simulink model "sampleModel1826"  (R2023a)
settings: Solver=VariableStepAuto  StartTime=0.0  StopTime=10.0  RelTol=1e-3
libraries: hdlsllib x4
settings Model: Creator=user1  LastModifiedBy=user1

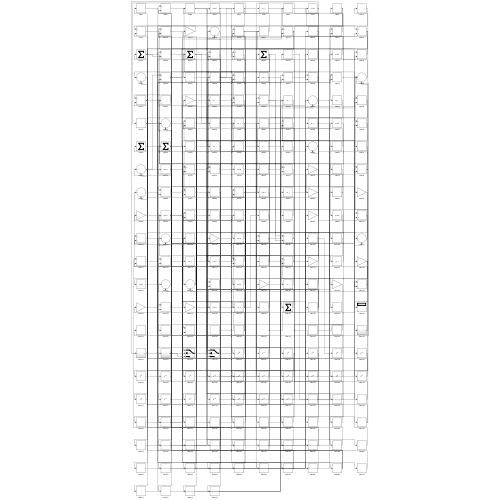
[thumbnail: Simulink's stored preview of the top-level diagram]
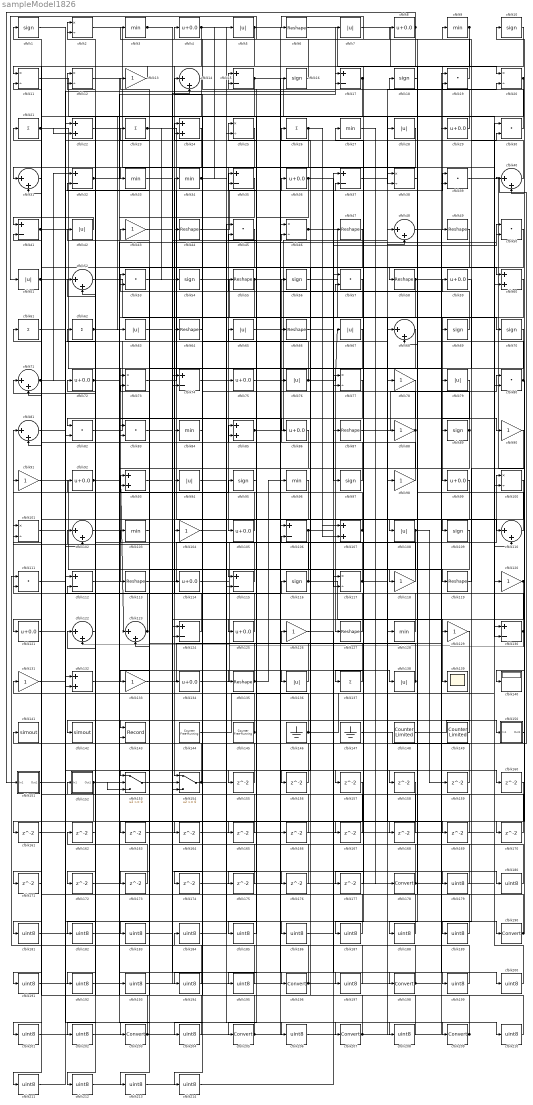
== system sampleModel1826 ==
  cfblk{1,10,16,18,54,56,69..70,89,95,97,109,116} (13 alike) : Signum
  cfblk{2,11..12,20,25,38,46,73,77,100..101,117} (12 alike) : Product  Inputs=*/  RndMeth=Zero  SaturateOnIntegerOverflow=on
  cfblk{14,31,40,48,52,68,71,81,102,110,122..123} (12 alike) : Sum  Inputs=|++
  cfblk{3,9,27,33..34,84,96,103,128} (9 alike) : MinMax
  cfblk{13,43,78,88,90..91,98,104,118,120,126,129,131,133} (14 alike) : Gain
  cfblk{4,8,29,36,59,72,75,86,92,99,105,114,121,125,134} (15 alike) : Bias  Bias=0.0  SaturateOnIntegerOverflow=off
  cfblk{15,17,32,35,37,41,74,106,112,115,124,130} (12 alike) : Sum  Inputs=+-
  cfblk{22,24,60,85,93,107,132} (7 alike) : Sum
  cfblk{5,7,28,42,51,63,65,67,76,79,94,108,136,138} (14 alike) : Abs  SaturateOnIntegerOverflow=off
  cfblk{19,30,39,45,50,53,57,80,82..83,111} (11 alike) : DotProduct  OutDataTypeStr=Inherit: Inherit via internal rule
  cfblk{6,44,47,49,55,58,64,66,87,113,119,127,135} (13 alike) : Reshape
  cfblk{21,23,26,61..62,137} (6 alike) : Sum  Inputs=+
  cfblk139 : Scope
  cfblk140 : Display
  cfblk141 : ToWorkspace  VariableName=simout  SaveFormat=Timeseries  SampleTime=-1
  cfblk142 : ToWorkspace  VariableName=simout  SaveFormat=Timeseries  SampleTime=-1
  cfblk143 : Record  FileSettingsInternal="{\"entries\":[{\"content\":{\"excelSettings\":{\"content\":{},\"type\":\"Streamout.ExcelSettings\"}},\"type\":\"Streamout.FileSettingStorage\",\"uuid\":\"\"}],\"packageUris\":[\"http:\\/\\/schema.mathworks.com\\/mf0\\/streamout_blocks\\/R2020a\"],\"version\":\"1.0\"}"  Layout=[1 1]  SignalsInternal="{\"entries\":[{\"content\":{\"signals\":[{\"content\":{\"blockPath\":[],\"dimensions\":[1],\"domain\":\"\",\"lineColor\":\"#a2142f\",\"plots\":[1],\"port\":1,\"signalID\":4356,\"signalName\":\"XY Graph:1\"},\"type\":\"RecordBlkView.Signal\",\"uuid\":\"\"},{\"content\":{\"blockPath\":[],\"dimensions\":[1],\"domain\":\"\",\"lineColor\":\"#139fff\",\"plots\":[1],\"port\":2,\"signalID\":4359,\"signalName\":\"XY Graph:2\"},\"type\":\"RecordBlkView.Signal\",\"uuid\":\"\"}]},\"type\":\"RecordBlkView.InputSignals\",\"uuid\":\"\"}],\"packageUris\":[\"http:\\/\\/schema.mathworks.com\\/mf0\\/streamout_blocks\\/R2020a\"],\"version\":\"1.0\"}"  VisualizationBindings="{\"xyplotplugin\":{\"info\":[{\"series\":[{\"bindingParametersList\":[{\"parameter\":\"X-Axis\",\"signalID\":4356,\"signalName\":\"XY Graph:1\"},{\"parameter\":\"Y-Axis\",\"signalID\":4359,\"signalName\":\"XY Graph:2\"}],\"seriesID\":47375}],\"subplotID\":1}]}}"  CompatibilityTag=XY  st=-1
  cfblk144 : hdlsllib/Sources/Counter Free-Running  NumBits=16  tsamp=-1
  cfblk145 : hdlsllib/Sources/Counter Free-Running  NumBits=16  tsamp=-1
  cfblk146 : Ground
  cfblk147 : Ground
  cfblk148 : hdlsllib/Sources/Counter Limited  uplimit=7  tsamp=-1
  cfblk149 : hdlsllib/Sources/Counter Limited  uplimit=7  tsamp=-1
  cfblk150 : Subsystem
      settings: LibrarySourceBlock=|
      | hdlsllib/Ports &
      | Subsystems/Subsystem
  cfblk151 : Subsystem
      settings: LibrarySourceBlock=|
      | hdlsllib/Ports &
      | Subsystems/Subsystem
  cfblk152 : Subsystem
      settings: LibrarySourceBlock=|
      | hdlsllib/Ports &
      | Subsystems/Subsystem
  cfblk153 : Switch  SaturateOnIntegerOverflow=off  InputSameDT=off
  cfblk154 : Switch  SaturateOnIntegerOverflow=off  InputSameDT=off
  cfblk{155..177} (23 alike) : Delay  SampleTime=1
  cfblk{178,190,196,198,203,205,207,209} (8 alike) : DataTypeConversion  SaturateOnIntegerOverflow=off  RndMeth=Floor
  cfblk{179..189,191..195,197,199..202,204,206,208,210..214} (29 alike) : DataTypeConversion  OutDataTypeStr=uint8  SaturateOnIntegerOverflow=off  RndMeth=Floor
  wires:
  cfblk105/1 -> cfblk81/1
  cfblk134/1 -> cfblk100/1
  cfblk154/1 -> cfblk141/1, cfblk160/1
  cfblk28/1 -> cfblk33/1
  cfblk17/1 -> cfblk63/1, cfblk185/1
  cfblk115/1 -> cfblk12/1
  cfblk73/1 -> cfblk36/1
  cfblk120/1 -> cfblk125/1, cfblk154/3
  cfblk97/1 -> cfblk21/1
  cfblk92/1 -> cfblk123/1, cfblk50/1
  cfblk109/1 -> cfblk143/1
  cfblk88/1 -> cfblk24/1, cfblk195/1
  cfblk69/1 -> cfblk53/1
  cfblk104/1 -> cfblk207/1
  cfblk55/1 -> cfblk163/1, cfblk199/1
  cfblk65/1 -> cfblk59/1
  cfblk130/1 -> cfblk91/1, cfblk122/2
  cfblk43/1 -> cfblk196/1
  cfblk117/1 -> cfblk72/1, cfblk169/1
  cfblk6/1 -> cfblk58/1
  cfblk5/1 -> cfblk25/2, cfblk167/1
  cfblk4/1 -> cfblk154/1, cfblk70/1
  cfblk2/1 -> cfblk105/1
  cfblk52/1 -> cfblk128/1
  cfblk136/1 -> cfblk35/1
  cfblk21/1 -> cfblk113/1, cfblk22/2
  cfblk16/1 -> cfblk51/1
  cfblk39/1 -> cfblk140/1
  cfblk106/1 -> cfblk133/1, cfblk50/2
  cfblk19/1 -> cfblk6/1
  cfblk35/1 -> cfblk143/2
  cfblk76/1 -> cfblk67/1, cfblk24/2
  cfblk23/1 -> cfblk109/1, cfblk54/1
  cfblk29/1 -> cfblk4/1
  cfblk125/1 -> cfblk34/1
  cfblk153/1 -> cfblk35/2
  cfblk27/1 -> cfblk178/1
  cfblk148/1 -> cfblk150/1(In1)
  cfblk108/1 -> cfblk154/2, cfblk159/1
  cfblk11/1 -> cfblk120/1
  cfblk149/1 -> cfblk142/1
  cfblk7/1 -> cfblk20/1
  cfblk146/1 -> cfblk85/1, cfblk80/2
  cfblk41/1 -> cfblk127/1, cfblk161/1
  cfblk116/1 -> cfblk139/1, cfblk71/1, cfblk115/1
  cfblk57/1 -> cfblk64/1
  cfblk10/1 -> cfblk49/1
  cfblk50/1 -> cfblk118/1
  cfblk30/1 -> cfblk7/1
  cfblk137/1 -> cfblk13/1
  cfblk51/1 -> cfblk129/1, cfblk30/2
  cfblk147/1 -> cfblk40/1
  cfblk82/1 -> cfblk38/1
  cfblk26/1 -> cfblk81/2, cfblk114/1, cfblk107/2
  cfblk66/1 -> cfblk37/1
  cfblk14/1 -> cfblk31/1
  cfblk85/1 -> cfblk28/1, cfblk158/1
  cfblk128/1 -> cfblk26/1
  cfblk145/1 -> cfblk93/1, cfblk11/2
  cfblk36/1 -> cfblk97/1, cfblk175/1
  cfblk9/1 -> cfblk82/2, cfblk201/1
  cfblk32/1 -> cfblk60/1, cfblk17/2
  cfblk95/1 -> cfblk15/1
  cfblk62/1 -> cfblk135/1, cfblk86/1
  cfblk46/1 -> cfblk99/1, cfblk107/1
  cfblk127/1 -> cfblk65/1
  cfblk111/1 -> cfblk37/2
  cfblk114/1 -> cfblk106/2
  cfblk54/1 -> cfblk100/2
  cfblk126/1 -> cfblk198/1
  cfblk70/1 -> cfblk124/2
  cfblk118/1 -> cfblk62/1
  cfblk12/1 -> cfblk138/1
  cfblk37/1 -> cfblk20/2
  cfblk22/1 -> cfblk130/2
  cfblk63/1 -> cfblk46/2
  cfblk3/1 -> cfblk136/1, cfblk115/2
  cfblk13/1 -> cfblk11/1
  cfblk131/1 -> cfblk39/1
  cfblk123/1 -> cfblk2/1, cfblk102/1
  cfblk138/1 -> cfblk55/1, cfblk25/1, cfblk32/2
  cfblk133/1 -> cfblk29/1
  cfblk60/1 -> cfblk153/1
  cfblk98/1 -> cfblk56/1
  cfblk44/1 -> cfblk19/1
  cfblk135/1 -> cfblk42/1, cfblk101/1, cfblk96/1
  cfblk64/1 -> cfblk94/1
  cfblk38/1 -> cfblk108/1
  cfblk89/1 -> cfblk93/2, cfblk8/1
  cfblk91/1 -> cfblk119/1
  cfblk113/1 -> cfblk60/2
  cfblk78/1 -> cfblk205/1
  cfblk79/1 -> cfblk82/1
  cfblk8/1 -> cfblk151/1(In1), cfblk177/1
  cfblk132/1 -> cfblk209/1
  cfblk121/1 -> cfblk66/1
  cfblk47/1 -> cfblk121/1
  cfblk152/1(Out1) -> cfblk95/1, cfblk153/3, cfblk171/1
  cfblk87/1 -> cfblk80/1
  cfblk119/1 -> cfblk9/1
  cfblk150/1(Out1) -> cfblk40/2
  cfblk15/1 -> cfblk38/2, cfblk110/1, cfblk71/2
  cfblk71/1 -> cfblk17/1, cfblk32/1
  cfblk107/1 -> cfblk84/1, cfblk137/1
  cfblk53/1 -> cfblk14/2
  cfblk58/1 -> cfblk90/1, cfblk153/2
  cfblk40/1 -> cfblk19/2
  cfblk151/1(Out1) -> cfblk116/1
  cfblk122/1 -> cfblk52/2
  cfblk56/1 -> cfblk88/1
  cfblk20/1 -> cfblk44/1, cfblk182/1
  cfblk80/1 -> cfblk3/1, cfblk170/1
  cfblk144/1 -> cfblk68/1
  cfblk59/1 -> cfblk79/1
  cfblk103/1 -> cfblk203/1
  cfblk124/1 -> cfblk23/1
  cfblk42/1 -> cfblk41/1
  cfblk34/1 -> cfblk75/1, cfblk5/1, cfblk117/2
  cfblk72/1 -> cfblk168/1, cfblk202/1
  cfblk74/1 -> cfblk190/1
  cfblk110/1 -> cfblk68/2
  cfblk81/1 -> cfblk155/1
  cfblk155/1 -> cfblk2/2
  cfblk49/1 -> cfblk156/1
  cfblk156/1 -> cfblk53/2
  cfblk33/1 -> cfblk157/1
  cfblk159/1 -> cfblk22/1
  cfblk161/1 -> cfblk102/2
  cfblk162/1 -> cfblk12/2
  cfblk163/1 -> cfblk110/2
  cfblk25/1 -> cfblk164/1
  cfblk164/1 -> cfblk106/1
  cfblk99/1 -> cfblk165/1
  cfblk165/1 -> cfblk1/1
  cfblk75/1 -> cfblk166/1
  cfblk166/1 -> cfblk31/2
  cfblk167/1 -> cfblk122/1
  cfblk168/1 -> cfblk117/1
  cfblk169/1 -> cfblk15/2
  cfblk170/1 -> cfblk73/2
  cfblk171/1 -> cfblk101/2
  cfblk24/1 -> cfblk172/1
  cfblk96/1 -> cfblk173/1
  cfblk173/1 -> cfblk52/1
  cfblk86/1 -> cfblk174/1
  cfblk174/1 -> cfblk130/1
  cfblk175/1 -> cfblk123/2
  cfblk93/1 -> cfblk176/1
  cfblk176/1 -> cfblk14/1
  cfblk177/1 -> cfblk57/2
  cfblk178/1 -> cfblk89/1, cfblk46/1
  cfblk94/1 -> cfblk179/1
  cfblk179/1 -> cfblk27/1
  cfblk83/1 -> cfblk180/1
  cfblk180/1 -> cfblk124/1
  cfblk158/1 -> cfblk181/1
  cfblk181/1 -> cfblk83/1
  cfblk182/1 -> cfblk83/2
  cfblk45/1 -> cfblk183/1
  cfblk183/1 -> cfblk134/1
  cfblk184/1 -> cfblk45/1
  cfblk185/1 -> cfblk45/2
  cfblk61/1 -> cfblk186/1
  cfblk186/1 -> cfblk87/1
  cfblk129/1 -> cfblk187/1
  cfblk187/1 -> cfblk61/1
  cfblk18/1 -> cfblk188/1
  cfblk188/1 -> cfblk131/1
  cfblk90/1 -> cfblk189/1
  cfblk189/1 -> cfblk18/1
  cfblk190/1 -> cfblk85/2, cfblk10/1
  cfblk100/1 -> cfblk191/1
  cfblk191/1 -> cfblk74/1
  cfblk157/1 -> cfblk192/1
  cfblk192/1 -> cfblk74/2
  cfblk112/1 -> cfblk193/1
  cfblk193/1 -> cfblk69/1
  cfblk160/1 -> cfblk194/1
  cfblk194/1 -> cfblk112/1
  cfblk195/1 -> cfblk112/2
  cfblk196/1 -> cfblk111/1, cfblk98/1
  cfblk102/1 -> cfblk197/1
  cfblk197/1 -> cfblk43/1
  cfblk198/1 -> cfblk162/1, cfblk41/2
  cfblk199/1 -> cfblk126/1
  cfblk48/1 -> cfblk200/1
  cfblk200/1 -> cfblk30/1
  cfblk201/1 -> cfblk48/1
  cfblk202/1 -> cfblk48/2
  cfblk203/1 -> cfblk111/2, cfblk16/1
  cfblk68/1 -> cfblk204/1
  cfblk204/1 -> cfblk103/1
  cfblk205/1 -> cfblk39/2, cfblk92/1
  cfblk1/1 -> cfblk206/1
  cfblk206/1 -> cfblk78/1
  cfblk207/1 -> cfblk76/1, cfblk152/1(In1)
  cfblk101/1 -> cfblk208/1
  cfblk208/1 -> cfblk104/1
  cfblk209/1 -> cfblk184/1, cfblk57/1, cfblk73/1
  cfblk172/1 -> cfblk210/1
  cfblk210/1 -> cfblk132/1
  cfblk31/1 -> cfblk211/1
  cfblk211/1 -> cfblk132/2
  cfblk77/1 -> cfblk212/1
  cfblk212/1 -> cfblk47/1
  cfblk67/1 -> cfblk213/1
  cfblk213/1 -> cfblk77/1
  cfblk84/1 -> cfblk214/1
  cfblk214/1 -> cfblk77/2

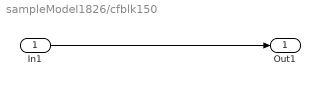
== system sampleModel1826/cfblk150 ==
  In1 : Inport
  Out1 : Outport
  wires:
  In1/1 -> Out1/1

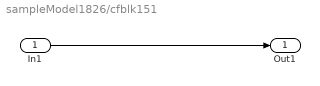
== system sampleModel1826/cfblk151 ==
  In1 : Inport
  Out1 : Outport
  wires:
  In1/1 -> Out1/1

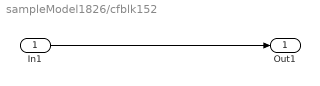
== system sampleModel1826/cfblk152 ==
  In1 : Inport
  Out1 : Outport
  wires:
  In1/1 -> Out1/1
